simulink library "ITKLib"  (R2022b)
settings: Solver=FixedStepDiscrete  StartTime=0.0  StopTime=10.0  FixedStep=0.01  RelTol=1e-3  EnableMultiTasking=on
values from neighbouring files (symbols this model uses):
  Glb_WhlRollgRd_SC = single(0.36)    [init_Global.m]
undefined symbols (not defined in the file or in its folder): docblock, SlDemoSign, SlDemoSign_Positive_SC, TaskTime_100ms_SC, TaskTime_10ms_SC, VehRefSpd_vMaxRefSpd_C
libraries: simulink x51, $bdroot x45, ITKLib_V14 x1
(part 6 of 10)

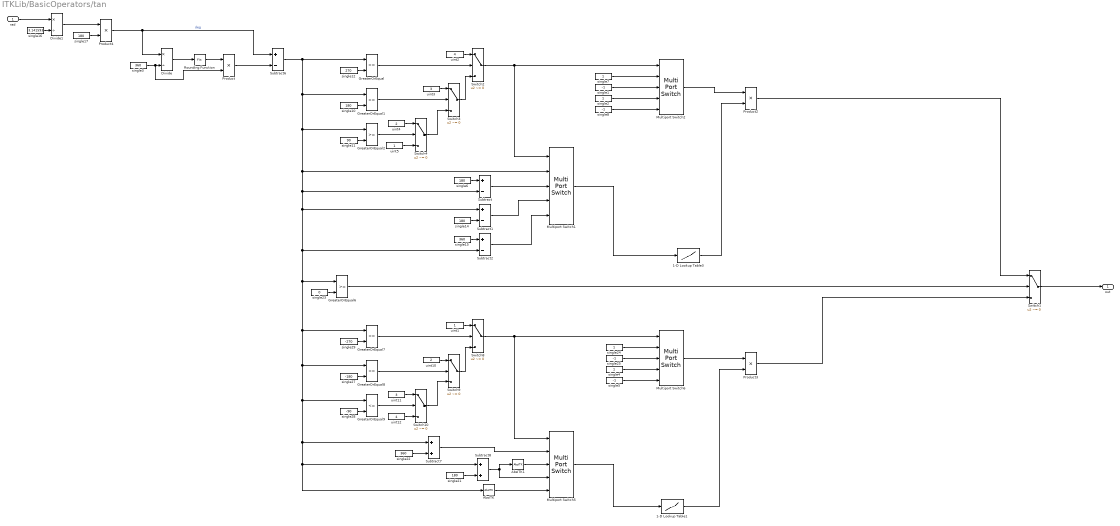
== system ITKLib/BasicOperators/tan ==
  rad : Inport
  1-D Lookup Table1 : Lookup_n-D  NumberOfTableDimensions=1  BreakpointsForDimension1=[0,5,10,15,20,25,30,35,40,45,50,55,60,65,70,75,80,85,89.9]  BreakpointsForDimension1DataTypeStr=single  Table=[0,0.0874886635259240,0.176326980708465,0.267949192431123,0.363970234266202,0.466307658154999,0.577350269189626,0.700207538209710,0.839099631177280,1.00000000000000,1.19175359259421,1.42814800674211,1.73205080756888,2.14450692050956,2.74747741945462,3.73205080756888,5.67128181961771,11.4300523027613,573]  TableDataTypeStr=single  IntermediateResultsDataTypeStr=single  ExtrapMethod=Clip  UseLastTableValue=on  InternalRulePriority=Speed  OutDataTypeStr=single  RndMeth=Simplest  FractionDataTypeStr=single
      settings: AttributesFormatString=|
      | input = %<BreakpointsForDimension1>
      | output = %<Table>
      | extrapolation-use end values: %<UseLastTableValue>
  1-D Lookup Table3 : Lookup_n-D  NumberOfTableDimensions=1  BreakpointsForDimension1=[0,5,10,15,20,25,30,35,40,45,50,55,60,65,70,75,80,85,89.9]  BreakpointsForDimension1DataTypeStr=single  Table=[0,0.0874886635259240,0.176326980708465,0.267949192431123,0.363970234266202,0.466307658154999,0.577350269189626,0.700207538209710,0.839099631177280,1.00000000000000,1.19175359259421,1.42814800674211,1.73205080756888,2.14450692050956,2.74747741945462,3.73205080756888,5.67128181961771,11.4300523027613,573]  TableDataTypeStr=single  IntermediateResultsDataTypeStr=single  ExtrapMethod=Clip  UseLastTableValue=on  InternalRulePriority=Speed  OutDataTypeStr=single  RndMeth=Simplest  FractionDataTypeStr=single
      settings: AttributesFormatString=|
      | input = %<BreakpointsForDimension1>
      | output = %<Table>
      | extrapolation-use end values: %<UseLastTableValue>
  AbsITK : $bdroot/BasicOperators/AbsITK
  AbsITK1 : $bdroot/BasicOperators/AbsITK
  Divide : Product  Inputs=*/  InputSameDT=on  RndMeth=Zero  SaturateOnIntegerOverflow=on
  Divide1 : Product  Inputs=*/  InputSameDT=on  RndMeth=Zero  SaturateOnIntegerOverflow=on
  GreaterOrEqual{,1..2,6} (4 alike) : RelationalOperator  OutDataTypeStr=boolean
  GreaterOrEqual7 : RelationalOperator  Operator=<=  OutDataTypeStr=boolean
  GreaterOrEqual8 : RelationalOperator  Operator=<=  OutDataTypeStr=boolean
  GreaterOrEqual9 : RelationalOperator  Operator=<=  OutDataTypeStr=boolean
  Multiport Switch{1..2,5..6} (4 alike) : MultiPortSwitch  Inputs=4  SaturateOnIntegerOverflow=off  InputSameDT=off
  Product{,2..4} (4 alike) : Product  InputSameDT=on  RndMeth=Zero  SaturateOnIntegerOverflow=on
  Rounding Function : Rounding  Operator=fix
  Subtract{,1..2,6} (4 alike) : Sum  Inputs=+-  InputSameDT=on  SaturateOnIntegerOverflow=on
  Subtract7 : Sum  InputSameDT=on  SaturateOnIntegerOverflow=on
  Subtract8 : Sum  InputSameDT=on  SaturateOnIntegerOverflow=on
  Switch{1..4,8..10} (7 alike) : Switch  Criteria=u2 ~= 0  SaturateOnIntegerOverflow=off  InputSameDT=off
      settings: AttributesFormatString=Criteria : %<Criteria>
  single{1,5,8,25} (4 alike) : Constant  Value=-1  OutDataTypeStr=single
      settings: AttributesFormatString=%<OutDataTypeStr>
  single{6,10,14,17,21} (5 alike) : Constant  Value=180  OutDataTypeStr=single
      settings: AttributesFormatString=%<OutDataTypeStr>
  single11 : Constant  Value=90  OutDataTypeStr=single
      settings: AttributesFormatString=%<OutDataTypeStr>
  single12 : Constant  Value=270  OutDataTypeStr=single
      settings: AttributesFormatString=%<OutDataTypeStr>
  single15 : Constant  Value=360  OutDataTypeStr=single
      settings: AttributesFormatString=%<OutDataTypeStr>
  single16 : Constant  Value=3.141593  OutDataTypeStr=single
      settings: AttributesFormatString=%<OutDataTypeStr>
  single{2,4,7,24} (4 alike) : Constant  OutDataTypeStr=single
      settings: AttributesFormatString=%<OutDataTypeStr>
  single22 : Constant  Value=360  OutDataTypeStr=single
      settings: AttributesFormatString=%<OutDataTypeStr>
  single23 : Constant  Value=0  OutDataTypeStr=single
      settings: AttributesFormatString=%<OutDataTypeStr>
  single27 : Constant  Value=-180  OutDataTypeStr=single
      settings: AttributesFormatString=%<OutDataTypeStr>
  single28 : Constant  Value=-90  OutDataTypeStr=single
      settings: AttributesFormatString=%<OutDataTypeStr>
  single29 : Constant  Value=-270  OutDataTypeStr=single
      settings: AttributesFormatString=%<OutDataTypeStr>
  single3 : Constant  Value=360  OutDataTypeStr=single
      settings: AttributesFormatString=%<OutDataTypeStr>
  uint1 : Constant  OutDataTypeStr=uint8
      settings: AttributesFormatString=%<OutDataTypeStr>
  uint10 : Constant  Value=2  OutDataTypeStr=uint8
      settings: AttributesFormatString=%<OutDataTypeStr>
  uint11 : Constant  Value=3  OutDataTypeStr=uint8
      settings: AttributesFormatString=%<OutDataTypeStr>
  uint12 : Constant  Value=4  OutDataTypeStr=uint8
      settings: AttributesFormatString=%<OutDataTypeStr>
  uint2 : Constant  Value=4  OutDataTypeStr=uint8
      settings: AttributesFormatString=%<OutDataTypeStr>
  uint3 : Constant  Value=3  OutDataTypeStr=uint8
      settings: AttributesFormatString=%<OutDataTypeStr>
  uint4 : Constant  Value=2  OutDataTypeStr=uint8
      settings: AttributesFormatString=%<OutDataTypeStr>
  uint5 : Constant  OutDataTypeStr=uint8
      settings: AttributesFormatString=%<OutDataTypeStr>
  out : Outport
  wires:
  uint3/1 -> Switch3/1
  uint10/1 -> Switch9/1
  single4/1 -> Multiport Switch6/4
  single1/1 -> Multiport Switch2/3
  Subtract7/1 -> Multiport Switch5/2
  Switch10/1 -> Switch9/3
  single29/1 -> GreaterOrEqual7/2
  Product2/1 -> Switch1/1
  GreaterOrEqual6/1 -> Switch1/2
  Divide/1 -> Rounding Function/1
  GreaterOrEqual8/1 -> Switch9/2
  single3/1 -> Product/2, Divide/2
  single22/1 -> Subtract7/2
  single21/1 -> Subtract8/2
  Switch3/1 -> Switch2/3
  GreaterOrEqual/1 -> Switch2/2
  uint2/1 -> Switch2/1
  Switch2/1 -> Multiport Switch1/1, Multiport Switch2/1
  Switch4/1 -> Switch3/3
  single6/1 -> Subtract/1
  single7/1 -> Multiport Switch2/2
  Subtract/1 -> Multiport Switch1/3
  uint4/1 -> Switch4/1
  single11/1 -> GreaterOrEqual2/2
  Multiport Switch2/1 -> Product2/1
  uint5/1 -> Switch4/3
  Subtract1/1 -> Multiport Switch1/4
  Subtract2/1 -> Multiport Switch1/5
  single27/1 -> GreaterOrEqual8/2
  Multiport Switch1/1 -> 1-D Lookup Table3/1
  uint12/1 -> Switch10/3
  Product/1 -> Subtract6/2
  Switch1/1 -> out/1
  Subtract8/1 -> AbsITK1/1, Multiport Switch5/4
  Multiport Switch6/1 -> Product3/1
  Multiport Switch5/1 -> 1-D Lookup Table1/1
  Switch8/1 -> Multiport Switch5/1, Multiport Switch6/1
  Product4/1 -> Divide/1, Subtract6/1  "deg"
  GreaterOrEqual9/1 -> Switch10/2
  GreaterOrEqual7/1 -> Switch8/2
  single12/1 -> GreaterOrEqual/2
  single28/1 -> GreaterOrEqual9/2
  single25/1 -> Multiport Switch6/3
  single14/1 -> Subtract1/2
  single2/1 -> Multiport Switch2/4
  single24/1 -> Multiport Switch6/2
  Rounding Function/1 -> Product/1
  single15/1 -> Subtract2/1
  Subtract6/1 -> GreaterOrEqual6/1, AbsITK/1, Subtract8/1, Subtract7/1, GreaterOrEqual9/1, GreaterOrEqual8/1, GreaterOrEqual7/1, Subtract2/2, Subtract1/1, Subtract/2, Multiport Switch1/2, GreaterOrEqual2/1, GreaterOrEqual1/1, GreaterOrEqual/1
  GreaterOrEqual2/1 -> Switch4/2
  1-D Lookup Table1/1 -> Product3/2
  single23/1 -> GreaterOrEqual6/2
  GreaterOrEqual1/1 -> Switch3/2
  single10/1 -> GreaterOrEqual1/2
  single5/1 -> Multiport Switch6/5
  uint11/1 -> Switch10/1
  Product3/1 -> Switch1/3
  single8/1 -> Multiport Switch2/5
  Switch9/1 -> Switch8/3
  uint1/1 -> Switch8/1
  1-D Lookup Table3/1 -> Product2/2
  Divide1/1 -> Product4/1
  single17/1 -> Product4/2
  single16/1 -> Divide1/2
  rad/1 -> Divide1/1
  AbsITK/1 -> Multiport Switch5/5
  AbsITK1/1 -> Multiport Switch5/3

== system ITKLib/BitOperation/GetBitU16 ==
  Pos : Inport  OutDataTypeStr=uint8
  u : Inport  Port=2  OutDataTypeStr=uint16
  Greater : RelationalOperator  Operator=>  OutDataTypeStr=boolean
  MATLAB Function : MATLAB Function  TreatAsAtomicUnit=on
  MATLAB Function1 : MATLAB Function  TreatAsAtomicUnit=on
  Subtract : Sum  Inputs=+-  InputSameDT=on  SaturateOnIntegerOverflow=on
  uint1 : Constant  Value=15  OutDataTypeStr=uint8  SampleTime=-1
      settings: AttributesFormatString=%<OutDataTypeStr>
  uint2 : Constant  Value=2  OutDataTypeStr=uint8  SampleTime=-1
      settings: AttributesFormatString=%<OutDataTypeStr>
  uint32 : Constant  Value=0  OutDataTypeStr=uint16  SampleTime=-1
      settings: AttributesFormatString=%<OutDataTypeStr>
  uint8 : Constant  OutDataTypeStr=uint8  SampleTime=-1
      settings: AttributesFormatString=%<OutDataTypeStr>
  Out : Outport  OutDataTypeStr=boolean
  wires:
  u/1 -> MATLAB Function/1(u)
  Subtract/1 -> MATLAB Function/3(N)
  Pos/1 -> Subtract/2
  uint1/1 -> Subtract/1, MATLAB Function1/3(N)
  MATLAB Function1/1(y) -> Greater/1
  Greater/1 -> Out/1
  uint32/1 -> Greater/2
  MATLAB Function/1(y) -> MATLAB Function1/1(u)
  uint2/1 -> MATLAB Function1/2(mode)  "Shift Right Logical"
  uint8/1 -> MATLAB Function/2(mode)  "Shift Left Logical"

== system ITKLib/BitOperation/GetBitU32 ==
  Pos : Inport  OutDataTypeStr=uint8
  u : Inport  Port=2  OutDataTypeStr=uint32
  Greater : RelationalOperator  Operator=>  OutDataTypeStr=boolean
  MATLAB Function : MATLAB Function  TreatAsAtomicUnit=on
  MATLAB Function1 : MATLAB Function  TreatAsAtomicUnit=on
  Subtract : Sum  Inputs=+-  InputSameDT=on  SaturateOnIntegerOverflow=on
  uint1 : Constant  Value=31  OutDataTypeStr=uint8  SampleTime=-1
      settings: AttributesFormatString=%<OutDataTypeStr>
  uint2 : Constant  Value=2  OutDataTypeStr=uint8  SampleTime=-1
      settings: AttributesFormatString=%<OutDataTypeStr>
  uint3 : Constant  OutDataTypeStr=uint8  SampleTime=-1
      settings: AttributesFormatString=%<OutDataTypeStr>
  uint8 : Constant  Value=0  OutDataTypeStr=uint32  SampleTime=-1
      settings: AttributesFormatString=%<OutDataTypeStr>
  Out : Outport  OutDataTypeStr=boolean
  wires:
  MATLAB Function1/1(y) -> Greater/1
  Greater/1 -> Out/1
  uint8/1 -> Greater/2
  Pos/1 -> Subtract/2
  u/1 -> MATLAB Function/1(u)
  uint1/1 -> MATLAB Function1/3(N), Subtract/1
  Subtract/1 -> MATLAB Function/3(N)
  uint3/1 -> MATLAB Function/2(mode)  "Shift Left Logical"
  MATLAB Function/1(y) -> MATLAB Function1/1(u)
  uint2/1 -> MATLAB Function1/2(mode)  "Shift Right Logical"

== system ITKLib/BitOperation/GetBitU8 ==
  Pos : Inport  OutDataTypeStr=uint8
  u : Inport  Port=2  OutDataTypeStr=uint8
  Greater : RelationalOperator  Operator=>  OutDataTypeStr=boolean
  MATLAB Function : MATLAB Function  TreatAsAtomicUnit=on
  MATLAB Function1 : MATLAB Function  TreatAsAtomicUnit=on
  Subtract : Sum  Inputs=+-  InputSameDT=on  SaturateOnIntegerOverflow=on
  uint1 : Constant  Value=7  OutDataTypeStr=uint8  SampleTime=-1
      settings: AttributesFormatString=%<OutDataTypeStr>
  uint2 : Constant  Value=2  OutDataTypeStr=uint8  SampleTime=-1
      settings: AttributesFormatString=%<OutDataTypeStr>
  uint32 : Constant  Value=0  OutDataTypeStr=uint8  SampleTime=-1
      settings: AttributesFormatString=%<OutDataTypeStr>
  uint8 : Constant  OutDataTypeStr=uint8  SampleTime=-1
      settings: AttributesFormatString=%<OutDataTypeStr>
  Out : Outport  OutDataTypeStr=boolean
  wires:
  u/1 -> MATLAB Function/1(u)
  uint1/1 -> MATLAB Function1/3(N), Subtract/1
  MATLAB Function1/1(y) -> Greater/1
  Pos/1 -> Subtract/2
  uint32/1 -> Greater/2
  Greater/1 -> Out/1
  Subtract/1 -> MATLAB Function/3(N)
  uint8/1 -> MATLAB Function/2(mode)  "Shift Left Logical"
  MATLAB Function/1(y) -> MATLAB Function1/1(u)
  uint2/1 -> MATLAB Function1/2(mode)  "Shift Right Logical"

== system ITKLib/BitOperation/MaskAnd ==
  In : Inport
  Mask : Inport  Port=2
  AND : Logic  OutDataTypeStr=boolean
  Bitwise Operator : simulink/Logic and Bit Operations/Bitwise Operator  logicop=AND  UseBitMask=off  NumInputPorts=2  BitMask=bin2dec('11011001')  BitMaskRealWorld=Stored Integer
  Data Type Conversion4 : DataTypeConversion  OutDataTypeStr=uint32  RndMeth=Simplest  SaturateOnIntegerOverflow=off
  Data Type Conversion7 : DataTypeConversion  OutDataTypeStr=uint32  RndMeth=Simplest  SaturateOnIntegerOverflow=off
  Relational Operator : RelationalOperator  Operator===  OutDataTypeStr=boolean  InputSameDT=off
  Relational Operator1 : RelationalOperator  Operator=~=  OutDataTypeStr=boolean  InputSameDT=off
  uint32 : Constant  Value=0  OutDataTypeStr=uint32  SampleTime=-1
      settings: AttributesFormatString=%<OutDataTypeStr>
  Out : Outport
  wires:
  Mask/1 -> Data Type Conversion4/1
  In/1 -> Data Type Conversion7/1
  AND/1 -> Out/1
  Bitwise Operator/1 -> Relational Operator/2
  Data Type Conversion7/1 -> Bitwise Operator/2
  Data Type Conversion4/1 -> Bitwise Operator/1, Relational Operator1/1, Relational Operator/1
  uint32/1 -> Relational Operator1/2
  Relational Operator1/1 -> AND/1
  Relational Operator/1 -> AND/2

== system ITKLib/BitOperation/MaskOr ==
  In : Inport
  Mask : Inport  Port=2
  Bitwise Operator : simulink/Logic and Bit Operations/Bitwise Operator  logicop=AND  UseBitMask=off  NumInputPorts=2  BitMask=bin2dec('11011001')  BitMaskRealWorld=Stored Integer
  DataTypeConversion : DataTypeConversion  OutDataTypeStr=uint32  SaturateOnIntegerOverflow=off  RndMeth=Floor
  DataTypeConversion1 : DataTypeConversion  OutDataTypeStr=uint32  SaturateOnIntegerOverflow=off  RndMeth=Floor
  DataTypeConversion2 : DataTypeConversion  OutDataTypeStr=uint32  SaturateOnIntegerOverflow=off  RndMeth=Floor
  Greater : RelationalOperator  OutDataTypeStr=boolean
  uint32 : Constant  OutDataTypeStr=uint32
      settings: AttributesFormatString=%<OutDataTypeStr>
  Out : Outport
  wires:
  Bitwise Operator/1 -> DataTypeConversion2/1
  In/1 -> DataTypeConversion1/1
  Mask/1 -> DataTypeConversion/1
  DataTypeConversion/1 -> Bitwise Operator/2
  DataTypeConversion1/1 -> Bitwise Operator/1
  uint32/1 -> Greater/2
  Greater/1 -> Out/1
  DataTypeConversion2/1 -> Greater/1

== system ITKLib/BitOperation/Merge16bit2out ==
  bit0 : Inport  OutDataTypeStr=boolean
  bit1 : Inport  Port=2  OutDataTypeStr=boolean
  bit2 : Inport  Port=3  OutDataTypeStr=boolean
  bit3 : Inport  Port=4  OutDataTypeStr=boolean
  bit4 : Inport  Port=5  OutDataTypeStr=boolean
  bit5 : Inport  Port=6  OutDataTypeStr=boolean
  bit6 : Inport  Port=7  OutDataTypeStr=boolean
  bit7 : Inport  Port=8  OutDataTypeStr=boolean
  bit8 : Inport  Port=9  OutDataTypeStr=boolean
  bit9 : Inport  Port=10  OutDataTypeStr=boolean
  bit10 : Inport  Port=11  OutDataTypeStr=boolean
  bit11 : Inport  Port=12  OutDataTypeStr=boolean
  bit12 : Inport  Port=13  OutDataTypeStr=boolean
  bit13 : Inport  Port=14  OutDataTypeStr=boolean
  bit14 : Inport  Port=15  OutDataTypeStr=boolean
  bit15 : Inport  Port=16  OutDataTypeStr=boolean
  Add : Sum  Inputs=++++++++++++++++  InputSameDT=on  SaturateOnIntegerOverflow=on
  Data Type Conversion{1..17} (17 alike) : DataTypeConversion  OutDataTypeStr=uint16  SaturateOnIntegerOverflow=off  RndMeth=Floor
  Shift Arithmetic1 : ArithShift  BitShiftNumber=1  BitShiftDirection=Left
  Shift Arithmetic10 : ArithShift  BitShiftNumber=10  BitShiftDirection=Left
  Shift Arithmetic2 : ArithShift  BitShiftNumber=2  BitShiftDirection=Left
  Shift Arithmetic3 : ArithShift  BitShiftNumber=3  BitShiftDirection=Left
  Shift Arithmetic4 : ArithShift  BitShiftNumber=4  BitShiftDirection=Left
  Shift Arithmetic42 : ArithShift  BitShiftNumber=11  BitShiftDirection=Left
  Shift Arithmetic43 : ArithShift  BitShiftNumber=12  BitShiftDirection=Left
  Shift Arithmetic44 : ArithShift  BitShiftNumber=13  BitShiftDirection=Left
  Shift Arithmetic45 : ArithShift  BitShiftNumber=14  BitShiftDirection=Left
  Shift Arithmetic46 : ArithShift  BitShiftNumber=15  BitShiftDirection=Left
  Shift Arithmetic5 : ArithShift  BitShiftNumber=5  BitShiftDirection=Left
  Shift Arithmetic6 : ArithShift  BitShiftNumber=6  BitShiftDirection=Left
  Shift Arithmetic7 : ArithShift  BitShiftNumber=7  BitShiftDirection=Left
  Shift Arithmetic8 : ArithShift  BitShiftNumber=8  BitShiftDirection=Left
  Shift Arithmetic9 : ArithShift  BitShiftNumber=9  BitShiftDirection=Left
  out : Outport
  wires:
  Data Type Conversion2/1 -> out/1
  bit12/1 -> Data Type Conversion14/1
  Shift Arithmetic45/1 -> Add/15
  Data Type Conversion5/1 -> Shift Arithmetic3/1
  Data Type Conversion4/1 -> Shift Arithmetic2/1
  Data Type Conversion3/1 -> Shift Arithmetic1/1
  bit8/1 -> Data Type Conversion10/1
  bit4/1 -> Data Type Conversion6/1
  Shift Arithmetic5/1 -> Add/6
  Data Type Conversion14/1 -> Shift Arithmetic43/1
  Data Type Conversion1/1 -> Add/1
  Shift Arithmetic6/1 -> Add/7
  Data Type Conversion8/1 -> Shift Arithmetic6/1
  Shift Arithmetic10/1 -> Add/11
  Data Type Conversion13/1 -> Shift Arithmetic42/1
  Data Type Conversion12/1 -> Shift Arithmetic10/1
  Shift Arithmetic42/1 -> Add/12
  bit5/1 -> Data Type Conversion7/1
  Shift Arithmetic1/1 -> Add/2
  Data Type Conversion7/1 -> Shift Arithmetic5/1
  bit1/1 -> Data Type Conversion3/1
  Data Type Conversion9/1 -> Shift Arithmetic7/1
  bit15/1 -> Data Type Conversion17/1
  Shift Arithmetic2/1 -> Add/3
  Add/1 -> Data Type Conversion2/1
  Shift Arithmetic9/1 -> Add/10
  Shift Arithmetic46/1 -> Add/16
  Shift Arithmetic7/1 -> Add/8
  Shift Arithmetic43/1 -> Add/13
  Shift Arithmetic8/1 -> Add/9
  Shift Arithmetic4/1 -> Add/5
  bit0/1 -> Data Type Conversion1/1
  Shift Arithmetic3/1 -> Add/4
  bit6/1 -> Data Type Conversion8/1
  bit9/1 -> Data Type Conversion11/1
  Shift Arithmetic44/1 -> Add/14
  Data Type Conversion16/1 -> Shift Arithmetic45/1
  Data Type Conversion17/1 -> Shift Arithmetic46/1
  bit7/1 -> Data Type Conversion9/1
  Data Type Conversion11/1 -> Shift Arithmetic9/1
  bit10/1 -> Data Type Conversion12/1
  bit11/1 -> Data Type Conversion13/1
  bit13/1 -> Data Type Conversion15/1
  bit2/1 -> Data Type Conversion4/1
  bit14/1 -> Data Type Conversion16/1
  Data Type Conversion15/1 -> Shift Arithmetic44/1
  Data Type Conversion6/1 -> Shift Arithmetic4/1
  bit3/1 -> Data Type Conversion5/1
  Data Type Conversion10/1 -> Shift Arithmetic8/1

== system ITKLib/BitOperation/Merge20bit2out ==
  bit0 : Inport  OutDataTypeStr=boolean
  bit1 : Inport  Port=2  OutDataTypeStr=boolean
  bit2 : Inport  Port=3  OutDataTypeStr=boolean
  bit3 : Inport  Port=4  OutDataTypeStr=boolean
  bit4 : Inport  Port=5  OutDataTypeStr=boolean
  bit5 : Inport  Port=6  OutDataTypeStr=boolean
  bit6 : Inport  Port=7  OutDataTypeStr=boolean
  bit7 : Inport  Port=8  OutDataTypeStr=boolean
  bit8 : Inport  Port=9  OutDataTypeStr=boolean
  bit9 : Inport  Port=10  OutDataTypeStr=boolean
  bit10 : Inport  Port=11  OutDataTypeStr=boolean
  bit11 : Inport  Port=12  OutDataTypeStr=boolean
  bit12 : Inport  Port=13  OutDataTypeStr=boolean
  bit13 : Inport  Port=14  OutDataTypeStr=boolean
  bit14 : Inport  Port=15  OutDataTypeStr=boolean
  bit15 : Inport  Port=16  OutDataTypeStr=boolean
  bit16 : Inport  Port=17  OutDataTypeStr=boolean
  bit17 : Inport  Port=18  OutDataTypeStr=boolean
  bit18 : Inport  Port=19  OutDataTypeStr=boolean
  bit19 : Inport  Port=20  OutDataTypeStr=boolean
  Add : Sum  Inputs=20  InputSameDT=on  SaturateOnIntegerOverflow=on
  Data Type Conversion{1..17,26..29} (21 alike) : DataTypeConversion  OutDataTypeStr=uint32  SaturateOnIntegerOverflow=off  RndMeth=Floor
  Shift Arithmetic1 : ArithShift  BitShiftNumber=1  BitShiftDirection=Left
  Shift Arithmetic10 : ArithShift  BitShiftNumber=10  BitShiftDirection=Left
  Shift Arithmetic11 : ArithShift  BitShiftNumber=16  BitShiftDirection=Left
  Shift Arithmetic12 : ArithShift  BitShiftNumber=17  BitShiftDirection=Left
  Shift Arithmetic13 : ArithShift  BitShiftNumber=18  BitShiftDirection=Left
  Shift Arithmetic14 : ArithShift  BitShiftNumber=19  BitShiftDirection=Left
  Shift Arithmetic2 : ArithShift  BitShiftNumber=2  BitShiftDirection=Left
  Shift Arithmetic3 : ArithShift  BitShiftNumber=3  BitShiftDirection=Left
  Shift Arithmetic4 : ArithShift  BitShiftNumber=4  BitShiftDirection=Left
  Shift Arithmetic42 : ArithShift  BitShiftNumber=11  BitShiftDirection=Left
  Shift Arithmetic43 : ArithShift  BitShiftNumber=12  BitShiftDirection=Left
  Shift Arithmetic44 : ArithShift  BitShiftNumber=13  BitShiftDirection=Left
  Shift Arithmetic45 : ArithShift  BitShiftNumber=14  BitShiftDirection=Left
  Shift Arithmetic46 : ArithShift  BitShiftNumber=15  BitShiftDirection=Left
  Shift Arithmetic5 : ArithShift  BitShiftNumber=5  BitShiftDirection=Left
  Shift Arithmetic6 : ArithShift  BitShiftNumber=6  BitShiftDirection=Left
  Shift Arithmetic7 : ArithShift  BitShiftNumber=7  BitShiftDirection=Left
  Shift Arithmetic8 : ArithShift  BitShiftNumber=8  BitShiftDirection=Left
  Shift Arithmetic9 : ArithShift  BitShiftNumber=9  BitShiftDirection=Left
  out : Outport
  wires:
  bit9/1 -> Data Type Conversion11/1
  bit2/1 -> Data Type Conversion4/1
  Add/1 -> Data Type Conversion2/1
  Data Type Conversion9/1 -> Shift Arithmetic7/1
  Data Type Conversion17/1 -> Shift Arithmetic46/1
  Data Type Conversion26/1 -> Shift Arithmetic11/1
  Shift Arithmetic43/1 -> Add/13
  bit0/1 -> Data Type Conversion1/1
  Data Type Conversion14/1 -> Shift Arithmetic43/1
  Data Type Conversion6/1 -> Shift Arithmetic4/1
  bit3/1 -> Data Type Conversion5/1
  bit11/1 -> Data Type Conversion13/1
  bit10/1 -> Data Type Conversion12/1
  Data Type Conversion13/1 -> Shift Arithmetic42/1
  bit13/1 -> Data Type Conversion15/1
  bit14/1 -> Data Type Conversion16/1
  Data Type Conversion11/1 -> Shift Arithmetic9/1
  bit6/1 -> Data Type Conversion8/1
  Data Type Conversion29/1 -> Shift Arithmetic14/1
  bit1/1 -> Data Type Conversion3/1
  bit5/1 -> Data Type Conversion7/1
  Shift Arithmetic4/1 -> Add/5
  bit7/1 -> Data Type Conversion9/1
  Data Type Conversion7/1 -> Shift Arithmetic5/1
  Shift Arithmetic3/1 -> Add/4
  Data Type Conversion8/1 -> Shift Arithmetic6/1
  Shift Arithmetic7/1 -> Add/8
  Shift Arithmetic6/1 -> Add/7
  Shift Arithmetic46/1 -> Add/16
  Shift Arithmetic42/1 -> Add/12
  Data Type Conversion12/1 -> Shift Arithmetic10/1
  Shift Arithmetic2/1 -> Add/3
  Data Type Conversion15/1 -> Shift Arithmetic44/1
  Shift Arithmetic44/1 -> Add/14
  Shift Arithmetic45/1 -> Add/15
  bit19/1 -> Data Type Conversion29/1
  bit12/1 -> Data Type Conversion14/1
  Shift Arithmetic5/1 -> Add/6
  Data Type Conversion16/1 -> Shift Arithmetic45/1
  Data Type Conversion5/1 -> Shift Arithmetic3/1
  bit16/1 -> Data Type Conversion26/1
  Shift Arithmetic12/1 -> Add/18
  Shift Arithmetic10/1 -> Add/11
  bit4/1 -> Data Type Conversion6/1
  Data Type Conversion10/1 -> Shift Arithmetic8/1
  Data Type Conversion2/1 -> out/1
  bit18/1 -> Data Type Conversion28/1
  bit15/1 -> Data Type Conversion17/1
  Shift Arithmetic8/1 -> Add/9
  Shift Arithmetic1/1 -> Add/2
  Data Type Conversion27/1 -> Shift Arithmetic12/1
  bit17/1 -> Data Type Conversion27/1
  bit8/1 -> Data Type Conversion10/1
  Shift Arithmetic14/1 -> Add/20
  Data Type Conversion1/1 -> Add/1
  Shift Arithmetic9/1 -> Add/10
  Data Type Conversion28/1 -> Shift Arithmetic13/1
  Shift Arithmetic11/1 -> Add/17
  Shift Arithmetic13/1 -> Add/19
  Data Type Conversion3/1 -> Shift Arithmetic1/1
  Data Type Conversion4/1 -> Shift Arithmetic2/1

== system ITKLib/BitOperation/Merge2bit2out ==
  bit0 : Inport  OutDataTypeStr=boolean
  bit1 : Inport  Port=2  OutDataTypeStr=boolean
  Add : Sum  InputSameDT=on  SaturateOnIntegerOverflow=on
  Data Type Conversion1 : DataTypeConversion  OutDataTypeStr=uint8  SaturateOnIntegerOverflow=off  RndMeth=Floor
  Data Type Conversion2 : DataTypeConversion  OutDataTypeStr=uint8  SaturateOnIntegerOverflow=off  RndMeth=Floor
  Data Type Conversion3 : DataTypeConversion  OutDataTypeStr=uint8  SaturateOnIntegerOverflow=off  RndMeth=Floor
  Shift Arithmetic1 : ArithShift  BitShiftNumber=1  BitShiftDirection=Left
  out : Outport
  wires:
  Data Type Conversion3/1 -> Shift Arithmetic1/1
  Add/1 -> Data Type Conversion1/1
  Data Type Conversion2/1 -> Add/1
  bit1/1 -> Data Type Conversion3/1
  Shift Arithmetic1/1 -> Add/2
  bit0/1 -> Data Type Conversion2/1
  Data Type Conversion1/1 -> out/1

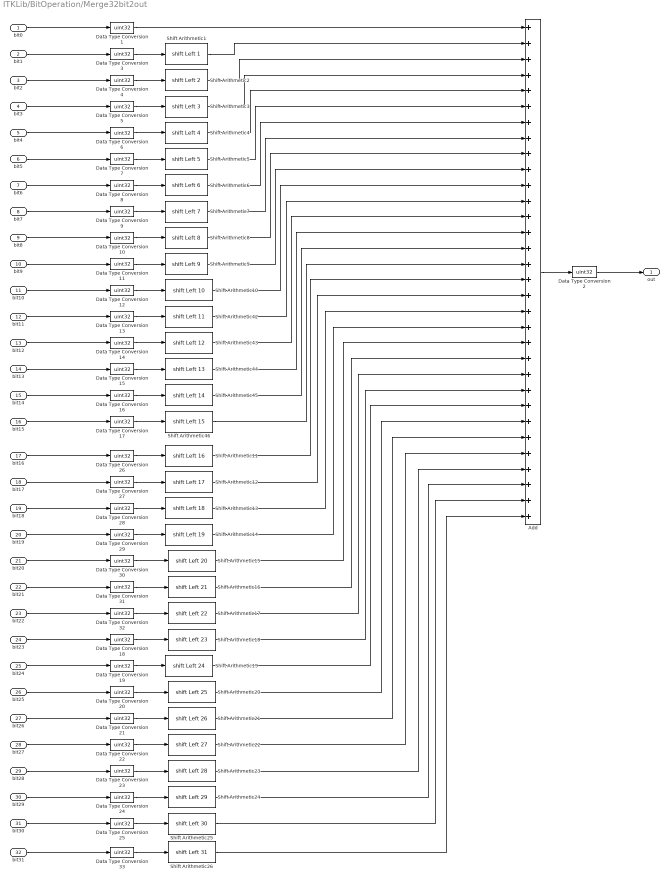
== system ITKLib/BitOperation/Merge32bit2out ==
  bit0 : Inport  OutDataTypeStr=boolean
  bit1 : Inport  Port=2  OutDataTypeStr=boolean
  bit2 : Inport  Port=3  OutDataTypeStr=boolean
  bit3 : Inport  Port=4  OutDataTypeStr=boolean
  bit4 : Inport  Port=5  OutDataTypeStr=boolean
  bit5 : Inport  Port=6  OutDataTypeStr=boolean
  bit6 : Inport  Port=7  OutDataTypeStr=boolean
  bit7 : Inport  Port=8  OutDataTypeStr=boolean
  bit8 : Inport  Port=9  OutDataTypeStr=boolean
  bit9 : Inport  Port=10  OutDataTypeStr=boolean
  bit10 : Inport  Port=11  OutDataTypeStr=boolean
  bit11 : Inport  Port=12  OutDataTypeStr=boolean
  bit12 : Inport  Port=13  OutDataTypeStr=boolean
  bit13 : Inport  Port=14  OutDataTypeStr=boolean
  bit14 : Inport  Port=15  OutDataTypeStr=boolean
  bit15 : Inport  Port=16  OutDataTypeStr=boolean
  bit16 : Inport  Port=17  OutDataTypeStr=boolean
  bit17 : Inport  Port=18  OutDataTypeStr=boolean
  bit18 : Inport  Port=19  OutDataTypeStr=boolean
  bit19 : Inport  Port=20  OutDataTypeStr=boolean
  bit20 : Inport  Port=21  OutDataTypeStr=boolean
  bit21 : Inport  Port=22  OutDataTypeStr=boolean
  bit22 : Inport  Port=23  OutDataTypeStr=boolean
  bit23 : Inport  Port=24  OutDataTypeStr=boolean
  bit24 : Inport  Port=25  OutDataTypeStr=boolean
  bit25 : Inport  Port=26  OutDataTypeStr=boolean
  bit26 : Inport  Port=27  OutDataTypeStr=boolean
  bit27 : Inport  Port=28  OutDataTypeStr=boolean
  bit28 : Inport  Port=29  OutDataTypeStr=boolean
  bit29 : Inport  Port=30  OutDataTypeStr=boolean
  bit30 : Inport  Port=31  OutDataTypeStr=boolean
  bit31 : Inport  Port=32  OutDataTypeStr=boolean
  Add : Sum  Inputs=32  InputSameDT=on  SaturateOnIntegerOverflow=on
  Data Type Conversion{1..33} (33 alike) : DataTypeConversion  OutDataTypeStr=uint32  SaturateOnIntegerOverflow=off  RndMeth=Floor
  Shift Arithmetic1 : ArithShift  BitShiftNumber=1  BitShiftDirection=Left
  Shift Arithmetic10 : ArithShift  BitShiftNumber=10  BitShiftDirection=Left
  Shift Arithmetic11 : ArithShift  BitShiftNumber=16  BitShiftDirection=Left
  Shift Arithmetic12 : ArithShift  BitShiftNumber=17  BitShiftDirection=Left
  Shift Arithmetic13 : ArithShift  BitShiftNumber=18  BitShiftDirection=Left
  Shift Arithmetic14 : ArithShift  BitShiftNumber=19  BitShiftDirection=Left
  Shift Arithmetic15 : ArithShift  BitShiftNumber=20  BitShiftDirection=Left
  Shift Arithmetic16 : ArithShift  BitShiftNumber=21  BitShiftDirection=Left
  Shift Arithmetic17 : ArithShift  BitShiftNumber=22  BitShiftDirection=Left
  Shift Arithmetic18 : ArithShift  BitShiftNumber=23  BitShiftDirection=Left
  Shift Arithmetic19 : ArithShift  BitShiftNumber=24  BitShiftDirection=Left
  Shift Arithmetic2 : ArithShift  BitShiftNumber=2  BitShiftDirection=Left
  Shift Arithmetic20 : ArithShift  BitShiftNumber=25  BitShiftDirection=Left
  Shift Arithmetic21 : ArithShift  BitShiftNumber=26  BitShiftDirection=Left
  Shift Arithmetic22 : ArithShift  BitShiftNumber=27  BitShiftDirection=Left
  Shift Arithmetic23 : ArithShift  BitShiftNumber=28  BitShiftDirection=Left
  Shift Arithmetic24 : ArithShift  BitShiftNumber=29  BitShiftDirection=Left
  Shift Arithmetic25 : ArithShift  BitShiftNumber=30  BitShiftDirection=Left
  Shift Arithmetic26 : ArithShift  BitShiftNumber=31  BitShiftDirection=Left
  Shift Arithmetic3 : ArithShift  BitShiftNumber=3  BitShiftDirection=Left
  Shift Arithmetic4 : ArithShift  BitShiftNumber=4  BitShiftDirection=Left
  Shift Arithmetic42 : ArithShift  BitShiftNumber=11  BitShiftDirection=Left
  Shift Arithmetic43 : ArithShift  BitShiftNumber=12  BitShiftDirection=Left
  Shift Arithmetic44 : ArithShift  BitShiftNumber=13  BitShiftDirection=Left
  Shift Arithmetic45 : ArithShift  BitShiftNumber=14  BitShiftDirection=Left
  Shift Arithmetic46 : ArithShift  BitShiftNumber=15  BitShiftDirection=Left
  Shift Arithmetic5 : ArithShift  BitShiftNumber=5  BitShiftDirection=Left
  Shift Arithmetic6 : ArithShift  BitShiftNumber=6  BitShiftDirection=Left
  Shift Arithmetic7 : ArithShift  BitShiftNumber=7  BitShiftDirection=Left
  Shift Arithmetic8 : ArithShift  BitShiftNumber=8  BitShiftDirection=Left
  Shift Arithmetic9 : ArithShift  BitShiftNumber=9  BitShiftDirection=Left
  out : Outport
  wires:
  Shift Arithmetic26/1 -> Add/32
  Shift Arithmetic25/1 -> Add/31
  Shift Arithmetic24/1 -> Add/30
  Shift Arithmetic23/1 -> Add/29
  Shift Arithmetic22/1 -> Add/28
  Shift Arithmetic21/1 -> Add/27
  Shift Arithmetic20/1 -> Add/26
  bit31/1 -> Data Type Conversion33/1
  Data Type Conversion33/1 -> Shift Arithmetic26/1
  Shift Arithmetic19/1 -> Add/25
  Shift Arithmetic18/1 -> Add/24
  Shift Arithmetic17/1 -> Add/23
  Shift Arithmetic16/1 -> Add/22
  Shift Arithmetic15/1 -> Add/21
  Shift Arithmetic14/1 -> Add/20
  Shift Arithmetic13/1 -> Add/19
  Shift Arithmetic12/1 -> Add/18
  Shift Arithmetic11/1 -> Add/17
  Data Type Conversion18/1 -> Shift Arithmetic18/1
  bit18/1 -> Data Type Conversion28/1
  Data Type Conversion29/1 -> Shift Arithmetic14/1
  Data Type Conversion23/1 -> Shift Arithmetic23/1
  bit29/1 -> Data Type Conversion24/1
  bit17/1 -> Data Type Conversion27/1
  bit28/1 -> Data Type Conversion23/1
  bit26/1 -> Data Type Conversion21/1
  bit25/1 -> Data Type Conversion20/1
  Data Type Conversion19/1 -> Shift Arithmetic19/1
  bit22/1 -> Data Type Conversion32/1
  Data Type Conversion25/1 -> Shift Arithmetic25/1
  Data Type Conversion24/1 -> Shift Arithmetic24/1
  bit24/1 -> Data Type Conversion19/1
  bit21/1 -> Data Type Conversion31/1
  bit30/1 -> Data Type Conversion25/1
  Data Type Conversion32/1 -> Shift Arithmetic17/1
  bit16/1 -> Data Type Conversion26/1
  Data Type Conversion30/1 -> Shift Arithmetic15/1
  bit20/1 -> Data Type Conversion30/1
  Data Type Conversion20/1 -> Shift Arithmetic20/1
  Data Type Conversion21/1 -> Shift Arithmetic21/1
  Data Type Conversion31/1 -> Shift Arithmetic16/1
  Data Type Conversion22/1 -> Shift Arithmetic22/1
  bit19/1 -> Data Type Conversion29/1
  bit23/1 -> Data Type Conversion18/1
  Data Type Conversion26/1 -> Shift Arithmetic11/1
  Data Type Conversion27/1 -> Shift Arithmetic12/1
  Data Type Conversion28/1 -> Shift Arithmetic13/1
  bit27/1 -> Data Type Conversion22/1
  Data Type Conversion2/1 -> out/1
  bit12/1 -> Data Type Conversion14/1
  Shift Arithmetic45/1 -> Add/15
  Data Type Conversion5/1 -> Shift Arithmetic3/1
  Data Type Conversion4/1 -> Shift Arithmetic2/1
  Data Type Conversion3/1 -> Shift Arithmetic1/1
  bit8/1 -> Data Type Conversion10/1
  bit4/1 -> Data Type Conversion6/1
  Shift Arithmetic5/1 -> Add/6
  Data Type Conversion14/1 -> Shift Arithmetic43/1
  Data Type Conversion1/1 -> Add/1
  Shift Arithmetic6/1 -> Add/7
  Data Type Conversion8/1 -> Shift Arithmetic6/1
  Shift Arithmetic10/1 -> Add/11
  Data Type Conversion13/1 -> Shift Arithmetic42/1
  Data Type Conversion12/1 -> Shift Arithmetic10/1
  Shift Arithmetic42/1 -> Add/12
  bit5/1 -> Data Type Conversion7/1
  Shift Arithmetic1/1 -> Add/2
  Data Type Conversion7/1 -> Shift Arithmetic5/1
  bit1/1 -> Data Type Conversion3/1
  Data Type Conversion9/1 -> Shift Arithmetic7/1
  bit15/1 -> Data Type Conversion17/1
  Shift Arithmetic2/1 -> Add/3
  Add/1 -> Data Type Conversion2/1
  Shift Arithmetic9/1 -> Add/10
  Shift Arithmetic46/1 -> Add/16
  Shift Arithmetic7/1 -> Add/8
  Shift Arithmetic43/1 -> Add/13
  Shift Arithmetic8/1 -> Add/9
  Shift Arithmetic4/1 -> Add/5
  bit0/1 -> Data Type Conversion1/1
  Shift Arithmetic3/1 -> Add/4
  bit6/1 -> Data Type Conversion8/1
  bit9/1 -> Data Type Conversion11/1
  Shift Arithmetic44/1 -> Add/14
  Data Type Conversion16/1 -> Shift Arithmetic45/1
  Data Type Conversion17/1 -> Shift Arithmetic46/1
  bit7/1 -> Data Type Conversion9/1
  Data Type Conversion11/1 -> Shift Arithmetic9/1
  bit10/1 -> Data Type Conversion12/1
  bit11/1 -> Data Type Conversion13/1
  bit13/1 -> Data Type Conversion15/1
  bit2/1 -> Data Type Conversion4/1
  bit14/1 -> Data Type Conversion16/1
  Data Type Conversion15/1 -> Shift Arithmetic44/1
  Data Type Conversion6/1 -> Shift Arithmetic4/1
  bit3/1 -> Data Type Conversion5/1
  Data Type Conversion10/1 -> Shift Arithmetic8/1

== system ITKLib/BitOperation/Merge3bit2out ==
  bit0 : Inport  OutDataTypeStr=boolean
  bit1 : Inport  Port=2  OutDataTypeStr=boolean
  bit2 : Inport  Port=3  OutDataTypeStr=boolean
  Add : Sum  Inputs=+++  InputSameDT=on  SaturateOnIntegerOverflow=on
  Data Type Conversion{1..4} (4 alike) : DataTypeConversion  OutDataTypeStr=uint8  SaturateOnIntegerOverflow=off  RndMeth=Floor
  Shift Arithmetic1 : ArithShift  BitShiftNumber=1  BitShiftDirection=Left
  Shift Arithmetic2 : ArithShift  BitShiftNumber=2  BitShiftDirection=Left
  out : Outport
  wires:
  Data Type Conversion3/1 -> Shift Arithmetic1/1
  Data Type Conversion4/1 -> Shift Arithmetic2/1
  Add/1 -> Data Type Conversion1/1
  bit2/1 -> Data Type Conversion4/1
  Shift Arithmetic2/1 -> Add/3
  Data Type Conversion2/1 -> Add/1
  bit1/1 -> Data Type Conversion3/1
  Shift Arithmetic1/1 -> Add/2
  bit0/1 -> Data Type Conversion2/1
  Data Type Conversion1/1 -> out/1

== system ITKLib/BitOperation/Merge4bit2out ==
  bit0 : Inport  OutDataTypeStr=boolean
  bit1 : Inport  Port=2  OutDataTypeStr=boolean
  bit2 : Inport  Port=3  OutDataTypeStr=boolean
  bit3 : Inport  Port=4  OutDataTypeStr=boolean
  Add : Sum  Inputs=++++  InputSameDT=on  SaturateOnIntegerOverflow=on
  Data Type Conversion{1..5} (5 alike) : DataTypeConversion  OutDataTypeStr=uint8  SaturateOnIntegerOverflow=off  RndMeth=Floor
  Shift Arithmetic1 : ArithShift  BitShiftNumber=1  BitShiftDirection=Left
  Shift Arithmetic2 : ArithShift  BitShiftNumber=2  BitShiftDirection=Left
  Shift Arithmetic3 : ArithShift  BitShiftNumber=3  BitShiftDirection=Left
  out : Outport
  wires:
  Data Type Conversion3/1 -> Shift Arithmetic1/1
  bit3/1 -> Data Type Conversion5/1
  Data Type Conversion4/1 -> Shift Arithmetic2/1
  Data Type Conversion5/1 -> Shift Arithmetic3/1
  Add/1 -> Data Type Conversion1/1
  bit2/1 -> Data Type Conversion4/1
  Shift Arithmetic2/1 -> Add/3
  Data Type Conversion2/1 -> Add/1
  Shift Arithmetic3/1 -> Add/4
  bit1/1 -> Data Type Conversion3/1
  Shift Arithmetic1/1 -> Add/2
  bit0/1 -> Data Type Conversion2/1
  Data Type Conversion1/1 -> out/1

== system ITKLib/BitOperation/Merge5bit2out ==
  bit0 : Inport  OutDataTypeStr=boolean
  bit1 : Inport  Port=2  OutDataTypeStr=boolean
  bit2 : Inport  Port=3  OutDataTypeStr=boolean
  bit3 : Inport  Port=4  OutDataTypeStr=boolean
  bit4 : Inport  Port=5  OutDataTypeStr=boolean
  Add : Sum  Inputs=+++++  InputSameDT=on  SaturateOnIntegerOverflow=on
  Data Type Conversion{1..6} (6 alike) : DataTypeConversion  OutDataTypeStr=uint8  SaturateOnIntegerOverflow=off  RndMeth=Floor
  Shift Arithmetic1 : ArithShift  BitShiftNumber=1  BitShiftDirection=Left
  Shift Arithmetic2 : ArithShift  BitShiftNumber=2  BitShiftDirection=Left
  Shift Arithmetic3 : ArithShift  BitShiftNumber=3  BitShiftDirection=Left
  Shift Arithmetic4 : ArithShift  BitShiftNumber=4  BitShiftDirection=Left
  out : Outport
  wires:
  bit4/1 -> Data Type Conversion6/1
  Data Type Conversion3/1 -> Shift Arithmetic1/1
  Data Type Conversion6/1 -> Shift Arithmetic4/1
  bit3/1 -> Data Type Conversion5/1
  Data Type Conversion4/1 -> Shift Arithmetic2/1
  Data Type Conversion5/1 -> Shift Arithmetic3/1
  Add/1 -> Data Type Conversion1/1
  bit2/1 -> Data Type Conversion4/1
  Shift Arithmetic2/1 -> Add/3
  Shift Arithmetic4/1 -> Add/5
  Data Type Conversion2/1 -> Add/1
  Shift Arithmetic3/1 -> Add/4
  bit1/1 -> Data Type Conversion3/1
  Shift Arithmetic1/1 -> Add/2
  bit0/1 -> Data Type Conversion2/1
  Data Type Conversion1/1 -> out/1

== system ITKLib/BitOperation/Merge6bit2out ==
  bit0 : Inport  OutDataTypeStr=boolean
  bit1 : Inport  Port=2  OutDataTypeStr=boolean
  bit2 : Inport  Port=3  OutDataTypeStr=boolean
  bit3 : Inport  Port=4  OutDataTypeStr=boolean
  bit4 : Inport  Port=5  OutDataTypeStr=boolean
  bit5 : Inport  Port=6  OutDataTypeStr=boolean
  Add : Sum  Inputs=++++++  InputSameDT=on  SaturateOnIntegerOverflow=on
  Data Type Conversion{1..7} (7 alike) : DataTypeConversion  OutDataTypeStr=uint8  SaturateOnIntegerOverflow=off  RndMeth=Floor
  Shift Arithmetic1 : ArithShift  BitShiftNumber=1  BitShiftDirection=Left
  Shift Arithmetic2 : ArithShift  BitShiftNumber=2  BitShiftDirection=Left
  Shift Arithmetic3 : ArithShift  BitShiftNumber=3  BitShiftDirection=Left
  Shift Arithmetic4 : ArithShift  BitShiftNumber=4  BitShiftDirection=Left
  Shift Arithmetic5 : ArithShift  BitShiftNumber=5  BitShiftDirection=Left
  out : Outport
  wires:
  bit4/1 -> Data Type Conversion6/1
  Shift Arithmetic5/1 -> Add/6
  Data Type Conversion3/1 -> Shift Arithmetic1/1
  Data Type Conversion6/1 -> Shift Arithmetic4/1
  bit3/1 -> Data Type Conversion5/1
  Data Type Conversion4/1 -> Shift Arithmetic2/1
  Data Type Conversion5/1 -> Shift Arithmetic3/1
  Add/1 -> Data Type Conversion1/1
  bit2/1 -> Data Type Conversion4/1
  Shift Arithmetic2/1 -> Add/3
  Shift Arithmetic4/1 -> Add/5
  Data Type Conversion2/1 -> Add/1
  Shift Arithmetic3/1 -> Add/4
  bit1/1 -> Data Type Conversion3/1
  bit5/1 -> Data Type Conversion7/1
  Shift Arithmetic1/1 -> Add/2
  bit0/1 -> Data Type Conversion2/1
  Data Type Conversion7/1 -> Shift Arithmetic5/1
  Data Type Conversion1/1 -> out/1

== system ITKLib/BitOperation/Merge7bit2out ==
  bit0 : Inport  OutDataTypeStr=boolean
  bit1 : Inport  Port=2  OutDataTypeStr=boolean
  bit2 : Inport  Port=3  OutDataTypeStr=boolean
  bit3 : Inport  Port=4  OutDataTypeStr=boolean
  bit4 : Inport  Port=5  OutDataTypeStr=boolean
  bit5 : Inport  Port=6  OutDataTypeStr=boolean
  bit6 : Inport  Port=7  OutDataTypeStr=boolean
  Add : Sum  Inputs=+++++++  InputSameDT=on  SaturateOnIntegerOverflow=on
  Data Type Conversion{1..8} (8 alike) : DataTypeConversion  OutDataTypeStr=uint8  SaturateOnIntegerOverflow=off  RndMeth=Floor
  Shift Arithmetic1 : ArithShift  BitShiftNumber=1  BitShiftDirection=Left
  Shift Arithmetic2 : ArithShift  BitShiftNumber=2  BitShiftDirection=Left
  Shift Arithmetic3 : ArithShift  BitShiftNumber=3  BitShiftDirection=Left
  Shift Arithmetic4 : ArithShift  BitShiftNumber=4  BitShiftDirection=Left
  Shift Arithmetic5 : ArithShift  BitShiftNumber=5  BitShiftDirection=Left
  Shift Arithmetic6 : ArithShift  BitShiftNumber=6  BitShiftDirection=Left
  out : Outport
  wires:
  bit4/1 -> Data Type Conversion6/1
  Shift Arithmetic5/1 -> Add/6
  Data Type Conversion3/1 -> Shift Arithmetic1/1
  Data Type Conversion6/1 -> Shift Arithmetic4/1
  bit3/1 -> Data Type Conversion5/1
  bit6/1 -> Data Type Conversion8/1
  Data Type Conversion4/1 -> Shift Arithmetic2/1
  Data Type Conversion5/1 -> Shift Arithmetic3/1
  Add/1 -> Data Type Conversion1/1
  bit2/1 -> Data Type Conversion4/1
  Shift Arithmetic2/1 -> Add/3
  Shift Arithmetic4/1 -> Add/5
  Data Type Conversion2/1 -> Add/1
  Shift Arithmetic3/1 -> Add/4
  bit1/1 -> Data Type Conversion3/1
  bit5/1 -> Data Type Conversion7/1
  Shift Arithmetic1/1 -> Add/2
  bit0/1 -> Data Type Conversion2/1
  Data Type Conversion7/1 -> Shift Arithmetic5/1
  Data Type Conversion8/1 -> Shift Arithmetic6/1
  Data Type Conversion1/1 -> out/1
  Shift Arithmetic6/1 -> Add/7

== system ITKLib/BitOperation/Merge8bit2out ==
  bit0 : Inport  OutDataTypeStr=boolean
  bit1 : Inport  Port=2  OutDataTypeStr=boolean
  bit2 : Inport  Port=3  OutDataTypeStr=boolean
  bit3 : Inport  Port=4  OutDataTypeStr=boolean
  bit4 : Inport  Port=5  OutDataTypeStr=boolean
  bit5 : Inport  Port=6  OutDataTypeStr=boolean
  bit6 : Inport  Port=7  OutDataTypeStr=boolean
  bit7 : Inport  Port=8  OutDataTypeStr=boolean
  Add : Sum  Inputs=++++++++  InputSameDT=on  SaturateOnIntegerOverflow=on
  Data Type Conversion{1..9} (9 alike) : DataTypeConversion  OutDataTypeStr=uint8  SaturateOnIntegerOverflow=off  RndMeth=Floor
  Shift Arithmetic1 : ArithShift  BitShiftNumber=1  BitShiftDirection=Left
  Shift Arithmetic2 : ArithShift  BitShiftNumber=2  BitShiftDirection=Left
  Shift Arithmetic3 : ArithShift  BitShiftNumber=3  BitShiftDirection=Left
  Shift Arithmetic4 : ArithShift  BitShiftNumber=4  BitShiftDirection=Left
  Shift Arithmetic5 : ArithShift  BitShiftNumber=5  BitShiftDirection=Left
  Shift Arithmetic6 : ArithShift  BitShiftNumber=6  BitShiftDirection=Left
  Shift Arithmetic7 : ArithShift  BitShiftNumber=7  BitShiftDirection=Left
  out : Outport
  wires:
  Data Type Conversion1/1 -> out/1
  Shift Arithmetic3/1 -> Add/4
  Shift Arithmetic2/1 -> Add/3
  Data Type Conversion7/1 -> Shift Arithmetic5/1
  bit0/1 -> Data Type Conversion2/1
  Data Type Conversion5/1 -> Shift Arithmetic3/1
  Data Type Conversion8/1 -> Shift Arithmetic6/1
  Shift Arithmetic6/1 -> Add/7
  Add/1 -> Data Type Conversion1/1
  Data Type Conversion9/1 -> Shift Arithmetic7/1
  Data Type Conversion4/1 -> Shift Arithmetic2/1
  Data Type Conversion6/1 -> Shift Arithmetic4/1
  Data Type Conversion3/1 -> Shift Arithmetic1/1
  bit1/1 -> Data Type Conversion3/1
  Shift Arithmetic1/1 -> Add/2
  Data Type Conversion2/1 -> Add/1
  Shift Arithmetic7/1 -> Add/8
  Shift Arithmetic4/1 -> Add/5
  bit3/1 -> Data Type Conversion5/1
  bit2/1 -> Data Type Conversion4/1
  bit7/1 -> Data Type Conversion9/1
  bit6/1 -> Data Type Conversion8/1
  bit5/1 -> Data Type Conversion7/1
  bit4/1 -> Data Type Conversion6/1
  Shift Arithmetic5/1 -> Add/6

== system ITKLib/BitOperation/Subsystem ==
  Pos : Inport
  BitVal : Inport  Port=2
  In : Inport  Port=3  OutDataTypeStr=uint8
  Bitwise Operator : simulink/Logic and Bit Operations/Bitwise Operator  logicop=OR  UseBitMask=on  BitMask=bin2dec('00000001')  BitMaskRealWorld=Stored Integer
  Bitwise Operator1 : simulink/Logic and Bit Operations/Bitwise Operator  logicop=AND  UseBitMask=on  BitMask=bin2dec('11111110')  BitMaskRealWorld=Stored Integer
  Bitwise Operator10 : simulink/Logic and Bit Operations/Bitwise Operator  logicop=OR  UseBitMask=on  BitMask=bin2dec('00100000')  BitMaskRealWorld=Stored Integer
  Bitwise Operator11 : simulink/Logic and Bit Operations/Bitwise Operator  logicop=AND  UseBitMask=on  BitMask=bin2dec('11011111')  BitMaskRealWorld=Stored Integer
  Bitwise Operator12 : simulink/Logic and Bit Operations/Bitwise Operator  logicop=OR  UseBitMask=on  BitMask=bin2dec('01000000')  BitMaskRealWorld=Stored Integer
  Bitwise Operator13 : simulink/Logic and Bit Operations/Bitwise Operator  logicop=AND  UseBitMask=on  BitMask=bin2dec('10111111')  BitMaskRealWorld=Stored Integer
  Bitwise Operator14 : simulink/Logic and Bit Operations/Bitwise Operator  logicop=OR  UseBitMask=on  BitMask=bin2dec('10000000')  BitMaskRealWorld=Stored Integer
  Bitwise Operator15 : simulink/Logic and Bit Operations/Bitwise Operator  logicop=AND  UseBitMask=on  BitMask=bin2dec('01111111')  BitMaskRealWorld=Stored Integer
  Bitwise Operator2 : simulink/Logic and Bit Operations/Bitwise Operator  logicop=OR  UseBitMask=on  BitMask=bin2dec('00000010')  BitMaskRealWorld=Stored Integer
  Bitwise Operator3 : simulink/Logic and Bit Operations/Bitwise Operator  logicop=AND  UseBitMask=on  BitMask=bin2dec('11111101')  BitMaskRealWorld=Stored Integer
  Bitwise Operator4 : simulink/Logic and Bit Operations/Bitwise Operator  logicop=OR  UseBitMask=on  BitMask=bin2dec('00000100')  BitMaskRealWorld=Stored Integer
  Bitwise Operator5 : simulink/Logic and Bit Operations/Bitwise Operator  logicop=AND  UseBitMask=on  BitMask=bin2dec('11111011')  BitMaskRealWorld=Stored Integer
  Bitwise Operator6 : simulink/Logic and Bit Operations/Bitwise Operator  logicop=OR  UseBitMask=on  BitMask=bin2dec('00001000')  BitMaskRealWorld=Stored Integer
  Bitwise Operator7 : simulink/Logic and Bit Operations/Bitwise Operator  logicop=AND  UseBitMask=on  BitMask=bin2dec('11110111')  BitMaskRealWorld=Stored Integer
  Bitwise Operator8 : simulink/Logic and Bit Operations/Bitwise Operator  logicop=OR  UseBitMask=on  BitMask=bin2dec('00010000')  BitMaskRealWorld=Stored Integer
  Bitwise Operator9 : simulink/Logic and Bit Operations/Bitwise Operator  logicop=AND  UseBitMask=on  BitMask=bin2dec('11101111')  BitMaskRealWorld=Stored Integer
  Multiport Switch : MultiPortSwitch  DataPortOrder=Zero-based contiguous  Inputs=8  DataPortForDefault=Additional data port  DiagnosticForDefault=Warning  zeroidx=on  OutDataTypeStr=uint8  InputSameDT=off
  Switch{1..8} (8 alike) : Switch  Criteria=u2 ~= 0  OutDataTypeStr=uint8  RndMeth=Simplest  InputSameDT=off
  Out : Outport  VectorParamsAs1DForOutWhenUnconnected=off
  wires:
  In/1 -> Multiport Switch/10, Bitwise Operator15/1, Bitwise Operator14/1, Bitwise Operator13/1, Bitwise Operator12/1, Bitwise Operator11/1, Bitwise Operator10/1, Bitwise Operator9/1, Bitwise Operator8/1, Bitwise Operator7/1, Bitwise Operator6/1, Bitwise Operator5/1, Bitwise Operator4/1, Bitwise Operator3/1, Bitwise Operator2/1, Bitwise Operator1/1, Bitwise Operator/1
  Bitwise Operator14/1 -> Switch8/1
  Bitwise Operator/1 -> Switch1/1
  Bitwise Operator6/1 -> Switch4/1
  BitVal/1 -> Switch7/2, Switch8/2, Switch6/2, Switch5/2, Switch4/2, Switch3/2, Switch2/2, Switch1/2
  Pos/1 -> Multiport Switch/1
  Bitwise Operator10/1 -> Switch6/1
  Bitwise Operator8/1 -> Switch5/1
  Bitwise Operator5/1 -> Switch3/3
  Switch6/1 -> Multiport Switch/7
  Bitwise Operator2/1 -> Switch2/1
  Switch3/1 -> Multiport Switch/4
  Bitwise Operator3/1 -> Switch2/3
  Switch8/1 -> Multiport Switch/9
  Switch7/1 -> Multiport Switch/8
  Switch2/1 -> Multiport Switch/3
  Bitwise Operator12/1 -> Switch7/1
  Switch1/1 -> Multiport Switch/2
  Bitwise Operator13/1 -> Switch7/3
  Bitwise Operator11/1 -> Switch6/3
  Bitwise Operator9/1 -> Switch5/3
  Switch5/1 -> Multiport Switch/6
  Bitwise Operator4/1 -> Switch3/1
  Multiport Switch/1 -> Out/1
  Switch4/1 -> Multiport Switch/5
  Bitwise Operator1/1 -> Switch1/3
  Bitwise Operator7/1 -> Switch4/3
  Bitwise Operator15/1 -> Switch8/3

== system ITKLib/BitOperation/Subsystem1 ==
  Pos : Inport
  In : Inport  Port=2  OutDataTypeStr=uint8
  Bitwise Operator : simulink/Logic and Bit Operations/Bitwise Operator  logicop=AND  UseBitMask=on  BitMask=bin2dec('00000001')  BitMaskRealWorld=Stored Integer
  Bitwise Operator10 : simulink/Logic and Bit Operations/Bitwise Operator  logicop=AND  UseBitMask=on  BitMask=bin2dec('00100000')  BitMaskRealWorld=Stored Integer
  Bitwise Operator12 : simulink/Logic and Bit Operations/Bitwise Operator  logicop=AND  UseBitMask=on  BitMask=bin2dec('01000000')  BitMaskRealWorld=Stored Integer
  Bitwise Operator14 : simulink/Logic and Bit Operations/Bitwise Operator  logicop=AND  UseBitMask=on  BitMask=bin2dec('10000000')  BitMaskRealWorld=Stored Integer
  Bitwise Operator2 : simulink/Logic and Bit Operations/Bitwise Operator  logicop=AND  UseBitMask=on  BitMask=bin2dec('00000010')  BitMaskRealWorld=Stored Integer
  Bitwise Operator4 : simulink/Logic and Bit Operations/Bitwise Operator  logicop=AND  UseBitMask=on  BitMask=bin2dec('00000100')  BitMaskRealWorld=Stored Integer
  Bitwise Operator6 : simulink/Logic and Bit Operations/Bitwise Operator  logicop=AND  UseBitMask=on  BitMask=bin2dec('00001000')  BitMaskRealWorld=Stored Integer
  Bitwise Operator8 : simulink/Logic and Bit Operations/Bitwise Operator  logicop=AND  UseBitMask=on  BitMask=bin2dec('00010000')  BitMaskRealWorld=Stored Integer
  Data Type Conversion{1..10} (10 alike) : DataTypeConversion  OutDataTypeStr=boolean  SaturateOnIntegerOverflow=off  RndMeth=Floor
  Multiport Switch : MultiPortSwitch  DataPortOrder=Zero-based contiguous  Inputs=8  DataPortForDefault=Additional data port  DiagnosticForDefault=Warning  zeroidx=on  OutDataTypeStr=uint8  InputSameDT=off
  Out : Outport  VectorParamsAs1DForOutWhenUnconnected=off
  wires:
  Data Type Conversion1/1 -> Multiport Switch/2
  Bitwise Operator/1 -> Data Type Conversion1/1
  Data Type Conversion5/1 -> Multiport Switch/6
  Bitwise Operator2/1 -> Data Type Conversion2/1
  Data Type Conversion6/1 -> Multiport Switch/7
  Bitwise Operator6/1 -> Data Type Conversion4/1
  Data Type Conversion2/1 -> Multiport Switch/3
  Bitwise Operator12/1 -> Data Type Conversion7/1
  Data Type Conversion10/1 -> Out/1
  Data Type Conversion3/1 -> Multiport Switch/4
  Data Type Conversion9/1 -> Multiport Switch/10
  Data Type Conversion7/1 -> Multiport Switch/8
  In/1 -> Bitwise Operator/1, Bitwise Operator2/1, Bitwise Operator4/1, Bitwise Operator6/1, Bitwise Operator8/1, Bitwise Operator10/1, Bitwise Operator12/1, Bitwise Operator14/1, Data Type Conversion9/1
  Bitwise Operator4/1 -> Data Type Conversion3/1
  Multiport Switch/1 -> Data Type Conversion10/1
  Pos/1 -> Multiport Switch/1
  Data Type Conversion4/1 -> Multiport Switch/5
  Bitwise Operator14/1 -> Data Type Conversion8/1
  Bitwise Operator8/1 -> Data Type Conversion5/1
  Bitwise Operator10/1 -> Data Type Conversion6/1
  Data Type Conversion8/1 -> Multiport Switch/9
